simulink model "prob1_214869"  (R2020a)
settings: Solver=VariableStepAuto  StartTime=0.0  StopTime=10.0  RelTol=1e-3
undefined symbols (not defined in the file): b, k1, k12, m1, m2
settings Model: Creator=sonal  LastModifiedBy=sonal

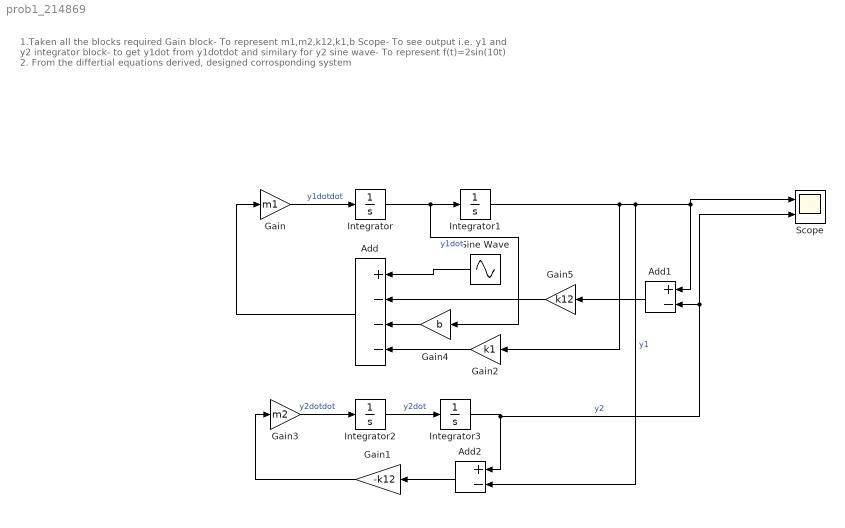
== system prob1_214869 ==
  note: 1.Taken all the blocks required
      | Gain block- To represent m1,m2,k12,k1,b
      | Scope- To see output i.e. y1 and y2
      | integrator block- to get y1dot from y1dotdot and similary for y2
      | sine wave- To represent f(t)=2sin(10t)
      |
      | 2. From the differtial equations derived, designed corrosponding system
  Add : Sum  Inputs=+---
  Add1 : Sum  Inputs=+-
  Add2 : Sum  Inputs=+-
  Gain : Gain  Gain=m1
  Gain1 : Gain  Gain=-k12
  Gain2 : Gain  Gain=k1
  Gain3 : Gain  Gain=m2
  Gain4 : Gain  Gain=b
  Gain5 : Gain  Gain=k12
  Integrator{,1..3} (4 alike) : Integrator
  Scope : Scope  NumInputPorts=2
  Sine Wave : Sin  Amplitude=2  Frequency=1.5915  SampleTime=0
  wires:
  Gain/1 -> Integrator/1  "y1dotdot"
  Integrator/1 -> Gain4/1, Integrator1/1  "y1dot"
  Sine Wave/1 -> Add/1
  Gain5/1 -> Add/2
  Add1/1 -> Gain5/1
  Integrator1/1 -> Gain2/1, Add2/2, Scope/1, Add1/1  "y1"
  Gain4/1 -> Add/3
  Gain2/1 -> Add/4
  Add/1 -> Gain/1
  Integrator2/1 -> Integrator3/1  "y2dot"
  Gain3/1 -> Integrator2/1  "y2dotdot"
  Integrator3/1 -> Scope/2, Add1/2, Add2/1  "y2"
  Add2/1 -> Gain1/1
  Gain1/1 -> Gain3/1
